simulink model "dng_pie"  (Simulink 6.0)
settings: Solver=ode45  StartTime=0.0  StopTime=inf  RelTol=1e-3
undefined symbols (not defined in the file or in its folder): slcm
libraries: dnglibv1 x4
settings Model: Creator=howie  LastModifiedBy=shaishaa
settings DataIOCC: SignalLoggingName=sigsOut
settings OptimizationCC: BooleanDataType=off  MultiInstanced=off
settings FormatCC: IgnoreBidirectionalLines=off
settings HardwareCC: TargetUnknown=on
settings CodeAppCC: FileBanners=off  CustomSymbols=off
settings GRTTargetCC: TargetFcnLib=iso_c_tmw.mat  IsERTTarget=off

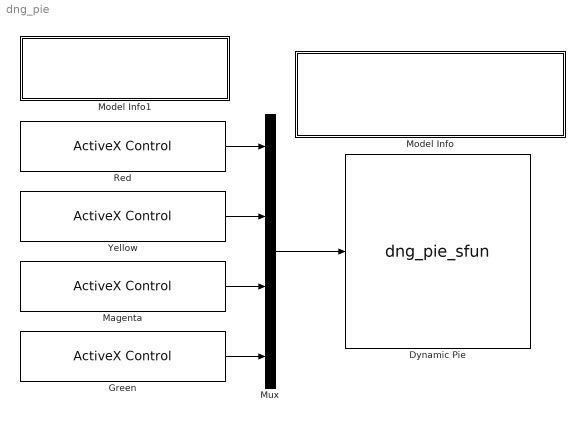
== system dng_pie ==
  Dynamic Pie : S-Function  Tag=000  LoadFcn=ax_block LoadFcn  FunctionName=dng_pie_sfun  Parameters=hActx  mask(ActiveX Block){progid=mwpercent.percentctrl.1, connect=input, input=, output=, dialOutEvent=, init=hActx.configuration='Percentage Indicator\Pie Charts\Dynamic Pie';, eventstr=, init_fcn=, update=, inblock=on, border=on, dialOut=0, parentList=, updateParam=0}
      mask prompts: progid "Program ID:"; connect "Connections:"; input "Input property:"; output "Output property:"; dialOutEvent "Event on which to output:"; init "Initialization command:"; eventstr "Other events and handlers:"; init_fcn "Handle location (function returning control handle or block name):"; update "Update command:"; inblock "In-block control"; dialOut "Dial Output Value:"
      mask help: Displays ActiveX control in model. Use block border to move/resize block. Right-click on block to edit properties. This block works only on Windows platforms.
      mask init:
      | str=sprintf('(Initialization\nFailed');
      | [hActx,inputprops,outputprops,inblock,dialOut] = ax_block('ActiveXMaskInit',gcs,gcb);
      | if isempty( hActx ) | strcmp(inblock,'off')
      |   str = 'ActiveX';
      | else
      |   str = '';
      | end
      settings: CopyFcn=ax_block CopyFcn  DeleteFcn=ax_block('DeleteBlock',gcb);  UndoDeleteFcn=ax_block('UndeleteBlock',gcb);  ModelCloseFcn=ax_block('ModelClosing', gcb);  PreSaveFcn=ax_block('PreSaveFcn')  PostSaveFcn=ax_block('SaveBlockControl');  NameChangeFcn=ax_block('NameBlockChange',gcb);  OpenFcn=ax_block('OpenFcn',gcbh);  ParentCloseFcn=ax_block('DeleteControl',gcb);  MoveFcn=ax_block('MoveBlockControl',gcb);
      mask Help: evalc('dnghelp')
      mask StyleString: edit,popup(input|output|both|neither),edit,edit,edit,edit,edit,edit,edit,checkbox,checkbox,edit,edit,edit
      mask CallbackString: ax_block Dirty||||ax_block Dirty|ax_block Dirty|ax_block Dirty|ax_block Dirty||ax_block('InBlockCallback');|ax_block('MoveBlockControl');|||
      mask Display: disp(str)
  Green : dnglibv1/ActiveX Control  progid=mwslider.sliderctrl.1  connect=output  output=Value  dialOutEvent=Slide Change  init=hActx.configuration='Slider\Basic\Horizontal\Simple Slider2';  inblock=on  border=on  dialOut=448.979591836735  updateParam=0
  Magenta : dnglibv1/ActiveX Control  progid=mwslider.sliderctrl.1  connect=output  output=Value  dialOutEvent=Slide Change  init=hActx.configuration='Slider\Basic\Horizontal\Simple Slider2';  inblock=on  border=on  dialOut=505.668934240363  updateParam=0
  Model Info : Subsystem  AncestorBlock=simulink/Model-Wide Utilities/Model Info  LoadFcn=slcm LoadBlock;  InitFcn=slcm('UpdateAllCMBlocksInThisModelInit')  mask(CMBlock){InitialSaveTempField=, InitialBlockCM=none, BlockCM=none, Frame=on, SaveTempField=, DisplayStringWithTags=|, MaskDisplayString=This model uses an S-function to manipulate\nthe portions of the Dynamic Pie block.\n\nIt normalizes the slider values to fill the pie., HorizontalTextAlignment=Left, LeftAlignmentValue=0.02, SourceBlockDiagram=dng_pie, TagMaxNumber=20, CMTag1=, CMTag2=, CMTag3=, CMTag4=, CMTag5=, CMTag6=, CMTag7=, CMTag8=, CMTag9=, CMTag10=, CMTag11=, CMTag12=, CMTag13=, CMTag14=, CMTag15=, CMTag16=, CMTag17=, CMTag18=, CMTag19=, CMTag20=}
      mask DisplayStringWithTags=|
      | This model uses an S-function to manipulate
      | the portions of the Dynamic Pie block.
      |
      | It normalizes the slider values to fill the pie.
      mask help: This block allows revision control information to be displayed within the model.
      settings: CopyFcn=slcm CopyBlock;  DeleteFcn=slcm Cancel;  PostSaveFcn=slcm('UpdateAllCMBlocksInThisModel')  NameChangeFcn=slcm Rename;  OpenFcn=slcm
      mask Display: text(str2num(LeftAlignmentValue), 0.5, MaskDisplayString, 'HorizontalAlignment', HorizontalTextAlignment)
  Model Info1 : Subsystem  AncestorBlock=simulink/Model-Wide Utilities/Model Info  LoadFcn=slcm LoadBlock;  InitFcn=slcm('UpdateAllCMBlocksInThisModelInit')  mask(CMBlock){InitialSaveTempField=, InitialBlockCM=none, BlockCM=none, Frame=on, SaveTempField=, DisplayStringWithTags=|, MaskDisplayString=Run the simulation and then\nmove the sliders with your mouse., HorizontalTextAlignment=Left, LeftAlignmentValue=0.02, SourceBlockDiagram=dng_pie, TagMaxNumber=20, CMTag1=, CMTag2=, CMTag3=, CMTag4=, CMTag5=, CMTag6=, CMTag7=, CMTag8=, CMTag9=, CMTag10=, CMTag11=, CMTag12=, CMTag13=, CMTag14=, CMTag15=, CMTag16=, CMTag17=, CMTag18=, CMTag19=, CMTag20=}
      mask DisplayStringWithTags=|
      | Run the simulation and then
      | move the sliders with your mouse.
      mask help: This block allows revision control information to be displayed within the model.
      settings: CopyFcn=slcm CopyBlock;  DeleteFcn=slcm Cancel;  PostSaveFcn=slcm('UpdateAllCMBlocksInThisModel')  NameChangeFcn=slcm Rename;  OpenFcn=slcm
      mask Display: text(str2num(LeftAlignmentValue), 0.5, MaskDisplayString, 'HorizontalAlignment', HorizontalTextAlignment)
  Mux : Mux
  Red : dnglibv1/ActiveX Control  progid=mwslider.sliderctrl.1  connect=output  output=Value  dialOutEvent=Slide Change  init=hActx.configuration='Slider\Basic\Horizontal\Simple Slider2';  inblock=on  border=on  dialOut=687.074829931973  updateParam=0
  Yellow : dnglibv1/ActiveX Control  progid=mwslider.sliderctrl.1  connect=output  output=Value  dialOutEvent=Slide Change  init=hActx.configuration='Slider\Basic\Horizontal\Simple Slider2';  inblock=on  border=on  dialOut=511.337868480726  updateParam=0
  wires:
  Mux/1 -> Dynamic Pie/1
  Red/1 -> Mux/1
  Yellow/1 -> Mux/2
  Magenta/1 -> Mux/3
  Green/1 -> Mux/4

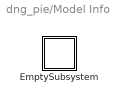
== system dng_pie/Model Info ==
  EmptySubsystem : Subsystem

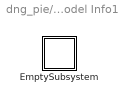
== system dng_pie/Model Info1 ==
  EmptySubsystem : Subsystem

== system dng_pie/Model Info/EmptySubsystem ==

== system dng_pie/Model Info1/EmptySubsystem ==
